simulink model "Simple_pendulum_simulation"  (R2023a)
settings: Solver=FixedStepAuto  StartTime=0.0  StopTime=10.0  FixedStep=1e-3  RelTol=1e-3
values from neighbouring files (symbols this model uses):
  b = 0.5    [simple_pendulum.m]
  g = 9.81    [simple_pendulum.m]
  l = 1    [simple_pendulum.m]
settings Model: Creator=mazen  LastModifiedBy=mazen

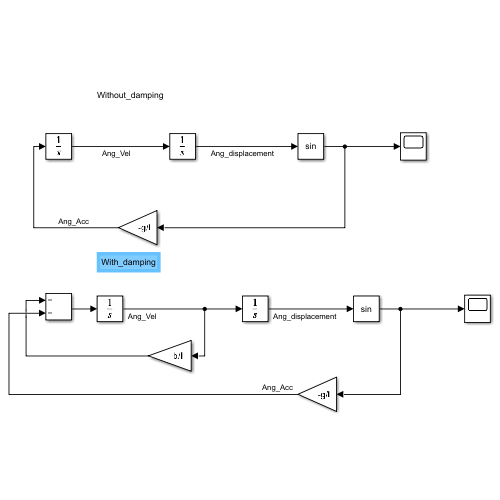
[thumbnail: Simulink's stored preview of the top-level diagram]
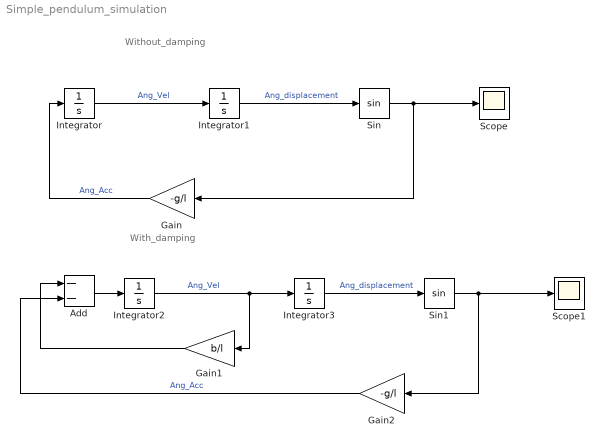
== system Simple_pendulum_simulation ==
  note: With_damping
  note: Without_damping
  Add : Sum  Inputs=--
  Gain : Gain  Gain=-g/l
  Gain1 : Gain  Gain=b/l
  Gain2 : Gain  Gain=-g/l
  Integrator : Integrator
  Integrator1 : Integrator  InitialCondition=2
  Integrator2 : Integrator
  Integrator3 : Integrator  InitialCondition=2
  Scope : Scope
  Scope1 : Scope
  Sin : Trigonometry
  Sin1 : Trigonometry
  wires:
  Integrator/1 -> Integrator1/1  "Ang_Vel"
  Integrator1/1 -> Sin/1  "Ang_displacement"
  Sin/1 -> Scope/1, Gain/1
  Gain/1 -> Integrator/1  "Ang_Acc"
  Integrator2/1 -> Gain1/1, Integrator3/1  "Ang_Vel"
  Integrator3/1 -> Sin1/1  "Ang_displacement"
  Sin1/1 -> Scope1/1, Gain2/1
  Gain1/1 -> Add/1
  Gain2/1 -> Add/2  "Ang_Acc"
  Add/1 -> Integrator2/1
